simulink model "simulink4"  (R2016a)
settings: Solver=ode23t  StartTime=0.0  StopTime=20.0  RelTol=1e-3
values from neighbouring files (symbols this model uses):
  g = 9.81    [pendulum.m]
  L1 = 0.800    (= 0.8)    [pendulum.m]
  L2 = 0.600    (= 0.6)    [pendulum.m]
  m1 = 0.500    (= 0.5)    [pendulum.m]
  m2 = 1.2    [pendulum.m]
  theta0 = pi/2    (= 1.57079632679)    [pendulum.m]
  theta02 = 0    [pendulum.m]
  v0 = 0    [pendulum.m]
undefined symbols (not defined in the file or in its folder): magnitude
settings Model: Creator=simone  LastModifiedBy=simone

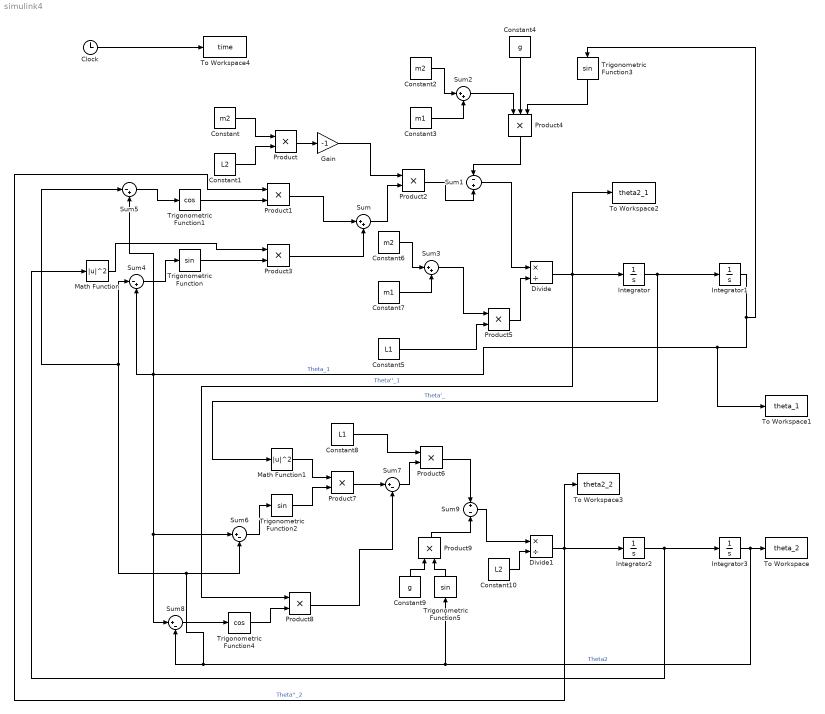
== system simulink4 ==
  Clock : Clock
  Constant : Constant  Value=m2
  Constant1 : Constant  Value=L2
  Constant10 : Constant  Value=L2
  Constant2 : Constant  Value=m2
  Constant3 : Constant  Value=m1
  Constant4 : Constant  Value=g
  Constant5 : Constant  Value=L1
  Constant6 : Constant  Value=m2
  Constant7 : Constant  Value=m1
  Constant8 : Constant  Value=L1
  Constant9 : Constant  Value=g
  Divide : Product  Inputs=*/
  Divide1 : Product  Inputs=*/
  Gain : Gain  Gain=-1
  Integrator : Integrator  InitialCondition=v0
  Integrator1 : Integrator  InitialCondition=theta0
  Integrator2 : Integrator  InitialCondition=v0
  Integrator3 : Integrator  InitialCondition=theta02
  Math Function : Math  Operator=magnitude^2  SaturateOnIntegerOverflow=on
  Math Function1 : Math  Operator=magnitude^2  SaturateOnIntegerOverflow=on
  Product{,1..3,5..9} (9 alike) : Product
  Product4 : Product  Inputs=3
  Sum : Sum  Inputs=|++
  Sum1 : Sum  Inputs=-|+
  Sum2 : Sum  Inputs=|++
  Sum3 : Sum  Inputs=|++
  Sum4 : Sum  Inputs=|-+
  Sum5 : Sum  Inputs=|-+
  Sum6 : Sum  Inputs=|+-
  Sum7 : Sum  Inputs=|+-
  Sum8 : Sum  Inputs=|+-
  Sum9 : Sum  Inputs=+-
  To Workspace : ToWorkspace  VariableName=theta_2  SaveFormat=Timeseries  SampleTime=-1
  To Workspace1 : ToWorkspace  VariableName=theta_1  SaveFormat=Timeseries  SampleTime=-1
  To Workspace2 : ToWorkspace  VariableName=theta2_1  SaveFormat=Timeseries  SampleTime=-1
  To Workspace3 : ToWorkspace  VariableName=theta2_2  SaveFormat=Timeseries  SampleTime=-1
  To Workspace4 : ToWorkspace  VariableName=time  SaveFormat=Timeseries  SampleTime=-1
  Trigonometric Function{,2..3,5} (4 alike) : Trigonometry
  Trigonometric Function1 : Trigonometry  Operator=cos
  Trigonometric Function4 : Trigonometry  Operator=cos
  wires:
  Constant/1 -> Product/1
  Constant1/1 -> Product/2
  Product/1 -> Gain/1
  Gain/1 -> Product2/1
  Product1/1 -> Sum/1
  Product3/1 -> Sum/2
  Sum/1 -> Product2/2
  Product2/1 -> Sum1/2
  Constant2/1 -> Sum2/1
  Constant3/1 -> Sum2/2
  Sum2/1 -> Product4/1
  Constant4/1 -> Product4/2
  Trigonometric Function3/1 -> Product4/3
  Product4/1 -> Sum1/1
  Sum1/1 -> Divide/1
  Constant6/1 -> Sum3/1
  Constant7/1 -> Sum3/2
  Sum3/1 -> Product5/1
  Constant5/1 -> Product5/2
  Product5/1 -> Divide/2
  Divide/1 -> To Workspace2/1, Product8/1, Integrator/1  "Theta''_1"
  Integrator/1 -> Math Function1/1, Integrator1/1  "Theta'_"
  Integrator1/1 -> Trigonometric Function3/1, To Workspace1/1, Sum8/1, Sum6/1, Sum4/2, Sum5/2  "Theta_1"
  Sum4/1 -> Trigonometric Function/1
  Sum5/1 -> Trigonometric Function1/1
  Trigonometric Function1/1 -> Product1/2
  Trigonometric Function/1 -> Product3/2
  Math Function/1 -> Product3/1
  Constant8/1 -> Product6/1
  Trigonometric Function2/1 -> Product7/2
  Math Function1/1 -> Product7/1
  Sum6/1 -> Trigonometric Function2/1
  Product7/1 -> Sum7/1
  Sum7/1 -> Product6/2
  Sum8/1 -> Trigonometric Function4/1
  Trigonometric Function4/1 -> Product8/2
  Product8/1 -> Sum7/2
  Product6/1 -> Sum9/1
  Product9/1 -> Sum9/2
  Constant9/1 -> Product9/1
  Trigonometric Function5/1 -> Product9/2
  Sum9/1 -> Divide1/1
  Constant10/1 -> Divide1/2
  Divide1/1 -> To Workspace3/1, Product1/1, Integrator2/1  "Theta''_2"
  Integrator2/1 -> Math Function/1, Integrator3/1
  Integrator3/1 -> Sum4/1, Sum5/1, Sum6/2, Sum8/2, Trigonometric Function5/1, To Workspace/1  "Theta2"
  Clock/1 -> To Workspace4/1
